simulink model "ebike2k8b"  (Simulink 7.2)
settings: Solver=ode3  StartTime=0.0  StopTime=0.5  FixedStep=0.001  MaxStep=0.001  MinStep=0.001  RelTol=1e-3
values from neighbouring files (symbols this model uses):
  A = 0.38    [run_sim.m]
  Cr = 0.003    [run_sim.m]
  Cw = 0.4    [run_sim.m]
  g = 9.8    [run_sim.m]
  M_Bike = 20    [run_sim.m]
  M_Driver = 60    [run_sim.m]
  P = 1.225    [run_sim.m]
libraries: simulink x3
settings Model: Creator=stwei  LastModifiedBy=kodm
settings DebuggingCC: StrictBusMsg=ErrorLevel1
settings CodeAppCC: CustomSymbolStrType=$N$R$M_T
settings GRTTargetCC: TargetFunctionLibrary=C89/C90 (ANSI)

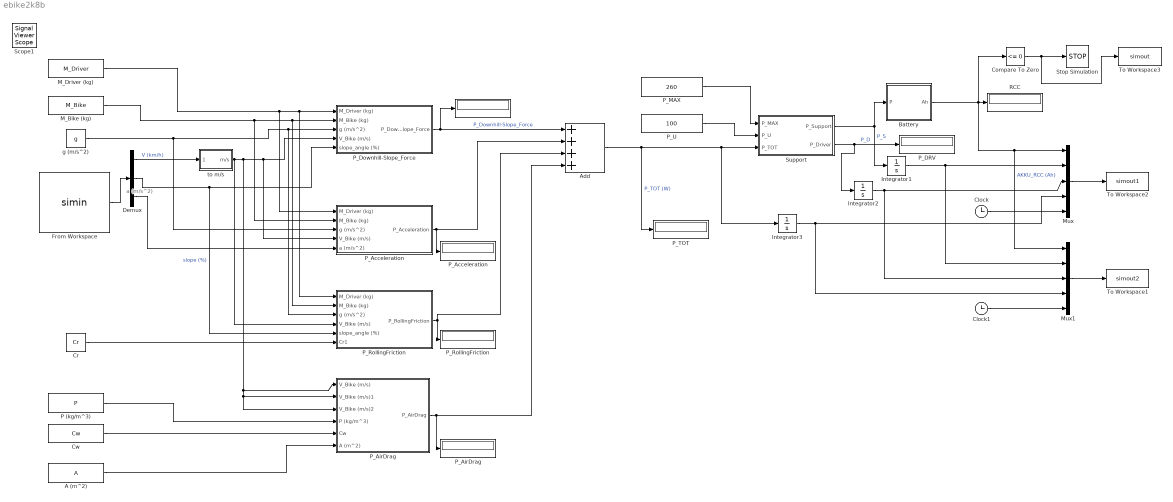
== system ebike2k8b ==
  note: a (m/s^2)
  "   " : Display
  "   P_Acceleration" : Display
  "   P_AirDrag" : Display
  "   P_RollingFriction" : Display
  " P_DRV" : Display
  " P_TOT" : Display
  A (m^2) : Constant  Value=A
  Add : Sum  Inputs=++++
  Battery : Subsystem
  Clock : Clock
  Clock1 : Clock
  Compare To Zero : simulink/Logic and Bit Operations/Compare To Zero  relop=<=  LogicOutDataTypeMode=boolean
  Cr : Constant  Value=Cr
  Cw : Constant  Value=Cw
  Demux : Demux  Outputs=3
  From Workspace : FromWorkspace  VariableName=simin  SampleTime=0  OutputAfterFinalValue=Setting to zero
  Integrator1 : Integrator
  Integrator2 : Integrator
  Integrator3 : Integrator
  M_Bike (kg) : Constant  Value=M_Bike
  M_Driver (kg) : Constant  Value=M_Driver
  Mux : Mux  Inputs=5
  Mux1 : Mux  Inputs=5
  P (kg/m^3) : Constant  Value=P
  P_Acceleration : Subsystem
  P_AirDrag : Subsystem
  P_Downhill-Slope_Force : Subsystem
  P_MAX : Constant  Value=260
  P_RollingFriction : Subsystem
  P_U : Constant  Value=100
  RCC : Display
  Stop Simulation : Stop
  Support : Subsystem
  To Workspace1 : ToWorkspace  VariableName=simout2  SaveFormat=Structure With Time  SampleTime=-1
  To Workspace2 : ToWorkspace  VariableName=simout1  SaveFormat=Structure With Time  SampleTime=-1
  To Workspace3 : ToWorkspace  VariableName=simout  SaveFormat=Structure With Time  SampleTime=-1
  g (m/s^2) : Constant  Value=g
  to m/s : Subsystem
  Scope1 : SignalViewerScope  IOType=viewer  NumInputPorts=9  ZoomMode=xonly  LegendLocations=|  RefreshTime=0.035000
      | 0.93194     0.94869     0.05625    0.018302
      | 0.89757     0.84158    0.090625    0.018302
      | 0.92075     0.73492    0.067708    0.018302
      |  0.9171     0.62871    0.071354    0.018302
      | 0.93325      0.5225    0.055208    0.018302
      | 0.92934     0.41674    0.058854    0.018302
      | 0.94757     0.31053    0.040625    0.018302
      | 0.94705     0.20432    0.041146    0.018302
      | 0.91684     0.09811    0.071354    0.018302
      settings: ShowLegends=on  TimeRange=2  YMin=0~0~0~0~9~-5~-5~-5~-5  YMax=1000~1000~1000~60~13~5~5~5~5
  wires:
  M_Driver (kg)/1 -> P_Acceleration/1(M_Driver (kg)), P_RollingFriction/1(M_Driver (kg)), P_Downhill-Slope_Force/1(M_Driver (kg))
  M_Bike (kg)/1 -> P_Acceleration/2(M_Bike (kg)), P_RollingFriction/2(M_Bike (kg)), P_Downhill-Slope_Force/2(M_Bike (kg))
  g (m/s^2)/1 -> P_Acceleration/3(g (m/s^2)), P_RollingFriction/3(g (m/s^2)), P_Downhill-Slope_Force/3(g (m/s^2))
  P_Downhill-Slope_Force/1(P_Downhill-Slope_Force) -> Add/1, "   "/1  "P_Downhill-Slope_Force"
  to m/s/1(m/s) -> P_RollingFriction/4(V_Bike (m/s)), P_AirDrag/3(V_Bike (m/s)2), P_AirDrag/2(V_Bike (m/s)1), P_AirDrag/1(V_Bike (m/s)), P_Acceleration/4(V_Bike (m/s)), P_Downhill-Slope_Force/4(V_Bike (m/s))
  Support/1(P_Support) -> Battery/1(P), Integrator1/1  "P_S"
  Support/2(P_Driver) -> Integrator2/1, " P_DRV"/1  "P_D"
  Battery/1(Ah) -> Compare To Zero/1, Mux1/1, Mux/1, RCC/1  "AKKU_RCC (Ah)"
  From Workspace/1 -> Demux/1
  Demux/1 -> to m/s/1(km/h)  "V (km/h)"
  Demux/2 -> P_RollingFriction/5(slope_angle (%)), P_Downhill-Slope_Force/5(slope_angle (%))  "slope (%)"
  P_Acceleration/1(P_Acceleration) -> "   P_Acceleration"/1, Add/2
  P_RollingFriction/1(P_RollingFriction) -> Add/3, "   P_RollingFriction"/1
  P_AirDrag/1(P_AirDrag) -> Add/4, "   P_AirDrag"/1
  Add/1 -> Integrator3/1, Support/3(P_TOT), " P_TOT"/1  "P_TOT (W)"
  Demux/3 -> P_Acceleration/5(a (m/s^2))
  P (kg/m^3)/1 -> P_AirDrag/4(P (kg/m^3))
  Cw/1 -> P_AirDrag/5(Cw)
  A (m^2)/1 -> P_AirDrag/6(A (m^2))
  Mux/1 -> To Workspace2/1
  P_U/1 -> Support/2(P_U)
  P_MAX/1 -> Support/1(P_MAX)
  Cr/1 -> P_RollingFriction/6(Cr1)
  Mux1/1 -> To Workspace1/1
  Integrator1/1 -> Mux1/2, Mux/2
  Integrator2/1 -> Mux1/3, Mux/3
  Integrator3/1 -> Mux1/4, Mux/4
  Clock/1 -> Mux/5
  Clock1/1 -> Mux1/5
  Compare To Zero/1 -> To Workspace3/1, Stop Simulation/1

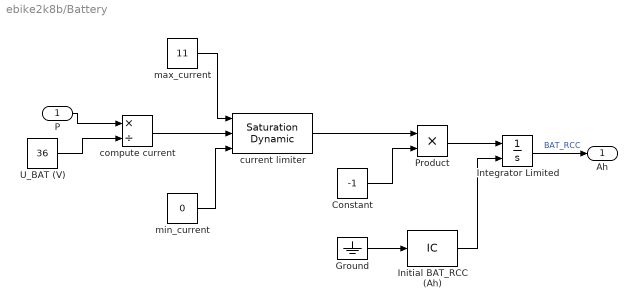
== system ebike2k8b/Battery ==
  P : Inport
  Constant : Constant  Value=-1
  Ground : Ground
  Initial BAT_RCC (Ah) : InitialCondition  Value=11
  Integrator Limited : Integrator  InitialConditionSource=external  LimitOutput=on  UpperSaturationLimit=13  LowerSaturationLimit=0
  Product : Product  RndMeth=Zero
  U_BAT (V) : Constant  Value=36
  compute current : Product  Inputs=*/
  current limiter : simulink/Discontinuities/Saturation Dynamic  OutMin=[]  OutMax=[]  OutDataTypeStr=Inherit: Same as second input  OutDataType=fixdt(1, 16)  OutScaling=2^-10  DoSatur=on
  max_current : Constant  Value=11
  min_current : Constant  Value=0
  Ah : Outport
  wires:
  Ground/1 -> Initial BAT_RCC (Ah)/1
  U_BAT (V)/1 -> compute current/2
  Initial BAT_RCC (Ah)/1 -> Integrator Limited/2
  Constant/1 -> Product/2
  Product/1 -> Integrator Limited/1
  P/1 -> compute current/1
  Integrator Limited/1 -> Ah/1  "BAT_RCC"
  current limiter/1 -> Product/1
  compute current/1 -> current limiter/2
  max_current/1 -> current limiter/1
  min_current/1 -> current limiter/3

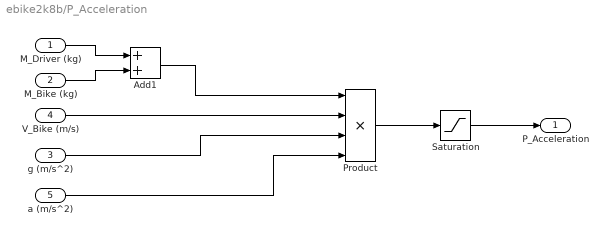
== system ebike2k8b/P_Acceleration ==
  M_Driver (kg) : Inport
  M_Bike (kg) : Inport  Port=2
  g (m/s^2) : Inport  Port=3
  V_Bike (m/s) : Inport  Port=4
  a (m/s^2) : Inport  Port=5
  Add1 : Sum
  Product : Product  Inputs=4  RndMeth=Zero
  Saturation : Saturate  UpperLimit=10000  LowerLimit=0
  P_Acceleration : Outport
  wires:
  Add1/1 -> Product/1
  M_Driver (kg)/1 -> Add1/1
  M_Bike (kg)/1 -> Add1/2
  V_Bike (m/s)/1 -> Product/2
  g (m/s^2)/1 -> Product/3
  Product/1 -> Saturation/1
  Saturation/1 -> P_Acceleration/1
  a (m/s^2)/1 -> Product/4

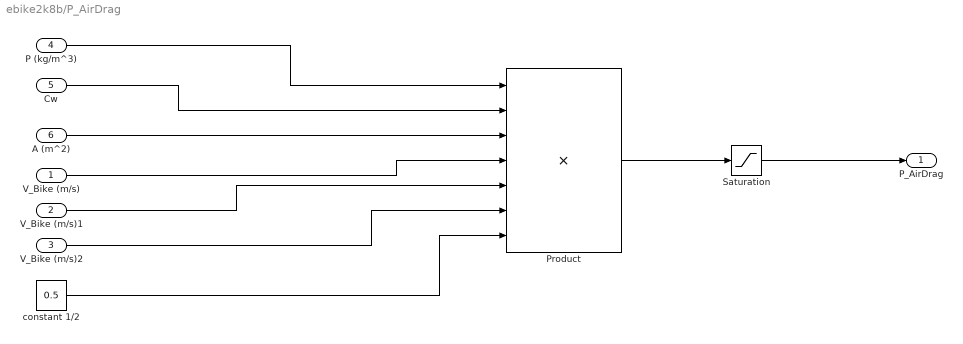
== system ebike2k8b/P_AirDrag ==
  V_Bike (m/s) : Inport
  V_Bike (m/s)1 : Inport  Port=2
  V_Bike (m/s)2 : Inport  Port=3
  P (kg/m^3) : Inport  Port=4
  Cw : Inport  Port=5
  A (m^2) : Inport  Port=6
  Product : Product  Inputs=7  RndMeth=Zero
  Saturation : Saturate  UpperLimit=10000  LowerLimit=0
  constant 1/2 : Constant  Value=0.5
  P_AirDrag : Outport
  wires:
  Product/1 -> Saturation/1
  Saturation/1 -> P_AirDrag/1
  V_Bike (m/s)/1 -> Product/4
  V_Bike (m/s)1/1 -> Product/5
  V_Bike (m/s)2/1 -> Product/6
  constant 1/2/1 -> Product/7
  P (kg/m^3)/1 -> Product/1
  Cw/1 -> Product/2
  A (m^2)/1 -> Product/3

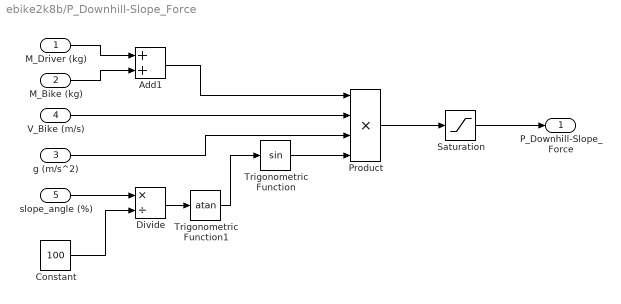
== system ebike2k8b/P_Downhill-Slope_Force ==
  M_Driver (kg) : Inport
  M_Bike (kg) : Inport  Port=2
  g (m/s^2) : Inport  Port=3
  V_Bike (m/s) : Inport  Port=4
  slope_angle (%) : Inport  Port=5
  Add1 : Sum
  Constant : Constant  Value=100
  Divide : Product  Inputs=*/
  Product : Product  Inputs=4  RndMeth=Zero
  Saturation : Saturate  UpperLimit=10000  LowerLimit=0
  Trigonometric Function : Trigonometry
  Trigonometric Function1 : Trigonometry  Operator=atan
  P_Downhill-Slope_Force : Outport
  wires:
  Add1/1 -> Product/1
  M_Driver (kg)/1 -> Add1/1
  M_Bike (kg)/1 -> Add1/2
  V_Bike (m/s)/1 -> Product/2
  g (m/s^2)/1 -> Product/3
  Trigonometric Function/1 -> Product/4
  Trigonometric Function1/1 -> Trigonometric Function/1
  slope_angle (%)/1 -> Divide/1
  Divide/1 -> Trigonometric Function1/1
  Constant/1 -> Divide/2
  Product/1 -> Saturation/1
  Saturation/1 -> P_Downhill-Slope_Force/1

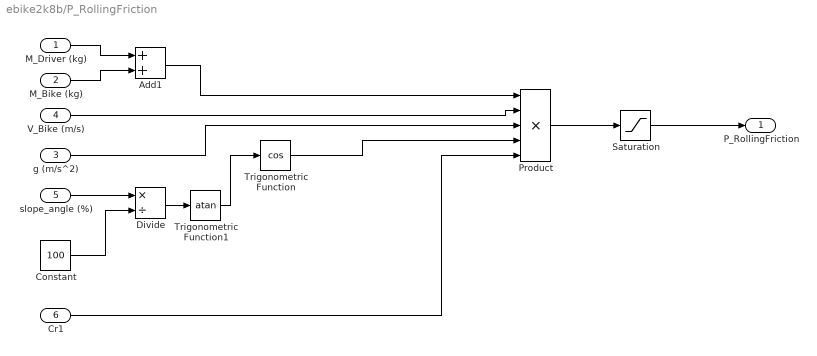
== system ebike2k8b/P_RollingFriction ==
  M_Driver (kg) : Inport
  M_Bike (kg) : Inport  Port=2
  g (m/s^2) : Inport  Port=3
  V_Bike (m/s) : Inport  Port=4
  slope_angle (%) : Inport  Port=5
  Cr1 : Inport  Port=6
  Add1 : Sum
  Constant : Constant  Value=100
  Divide : Product  Inputs=*/
  Product : Product  Inputs=5  RndMeth=Zero
  Saturation : Saturate  UpperLimit=10000  LowerLimit=0
  Trigonometric Function : Trigonometry  Operator=cos
  Trigonometric Function1 : Trigonometry  Operator=atan
  P_RollingFriction : Outport
  wires:
  Add1/1 -> Product/1
  M_Driver (kg)/1 -> Add1/1
  M_Bike (kg)/1 -> Add1/2
  V_Bike (m/s)/1 -> Product/2
  g (m/s^2)/1 -> Product/3
  Trigonometric Function/1 -> Product/4
  Trigonometric Function1/1 -> Trigonometric Function/1
  slope_angle (%)/1 -> Divide/1
  Divide/1 -> Trigonometric Function1/1
  Constant/1 -> Divide/2
  Product/1 -> Saturation/1
  Saturation/1 -> P_RollingFriction/1
  Cr1/1 -> Product/5

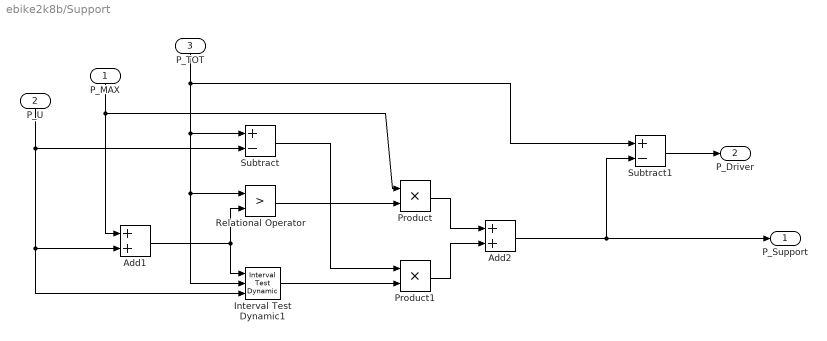
== system ebike2k8b/Support ==
  P_MAX : Inport  Orientation=down
  P_U : Inport  Orientation=down  Port=2
  P_TOT : Inport  Orientation=down  Port=3
  Add1 : Sum
  Add2 : Sum
  Interval Test Dynamic1 : simulink/Logic and Bit Operations/Interval Test Dynamic  IntervalClosedRight=on  IntervalClosedLeft=on  LogicOutDataTypeMode=uint8
  Product : Product  RndMeth=Zero
  Product1 : Product  RndMeth=Zero
  Relational Operator : RelationalOperator  Operator=>  OutDataTypeStr=boolean  LogicOutDataTypeMode=boolean
  Subtract : Sum  Inputs=+-
  Subtract1 : Sum  Inputs=+-
  P_Support : Outport
  P_Driver : Outport  Port=2
  wires:
  Add1/1 -> Interval Test Dynamic1/1, Relational Operator/2
  P_TOT/1 -> Subtract1/1, Subtract/1, Interval Test Dynamic1/2, Relational Operator/1
  P_U/1 -> Subtract/2, Interval Test Dynamic1/3, Add1/2
  P_MAX/1 -> Product/1, Add1/1
  Relational Operator/1 -> Product/2
  Subtract/1 -> Product1/1
  Interval Test Dynamic1/1 -> Product1/2
  Product/1 -> Add2/1
  Product1/1 -> Add2/2
  Add2/1 -> Subtract1/2, P_Support/1
  Subtract1/1 -> P_Driver/1

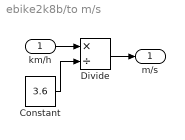
== system ebike2k8b/to m/s ==
  km/h : Inport
  Constant : Constant  Value=3.6
  Divide : Product  Inputs=*/
  m/s : Outport
  wires:
  Constant/1 -> Divide/2
  km/h/1 -> Divide/1
  Divide/1 -> m/s/1
